simulink model "purePursuit2"  (R2022a)
settings: Solver=VariableStepAuto  StartTime=0.0  StopTime=inf  RelTol=1e-3
undefined symbols (not defined in the file or in its folder): Angular, esc, hz, L, ld, Linear, path
libraries: robotlib x3, dspstat3 x1
settings Model: Creator=kisho  LastModifiedBy=kishor
settings DebuggingCC: UnconnectedInputMsg=warning  UnconnectedOutputMsg=warning  UnconnectedLineMsg=warning
settings RTWCC: DLArmComputeVersion=19.05

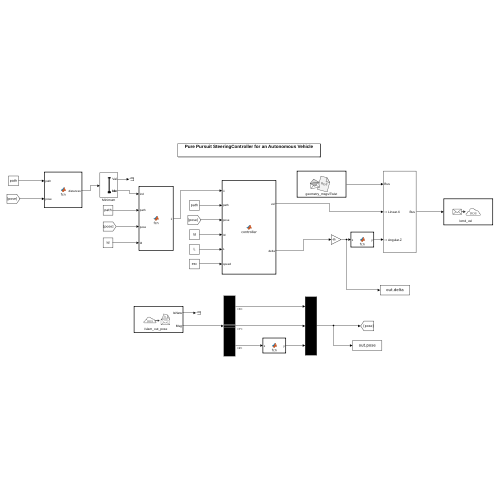
[thumbnail: Simulink's stored preview of the top-level diagram]
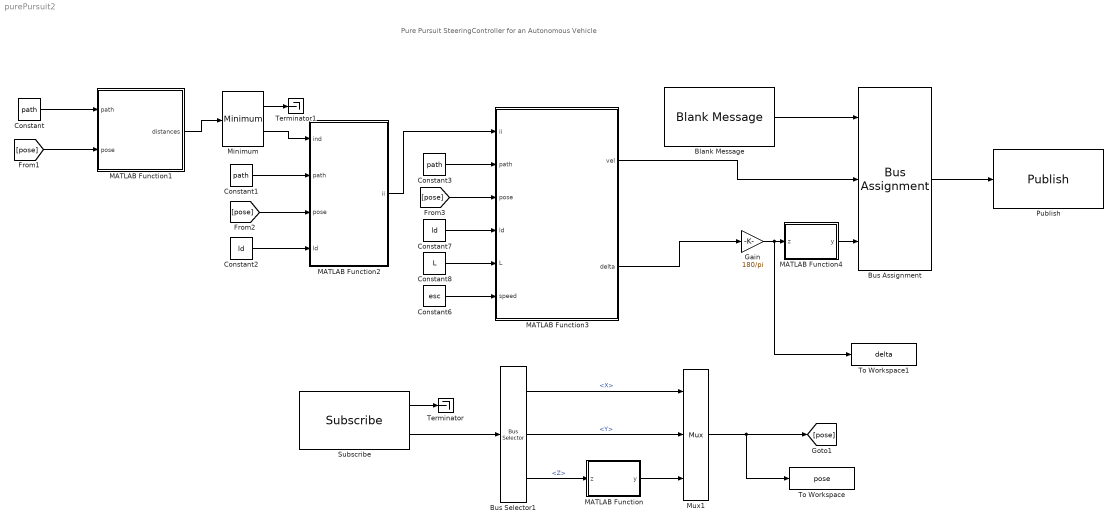
== system purePursuit2 ==
  note: Pure Pursuit SteeringController for an Autonomous Vehicle
  Blank Message : robotlib/Blank Message  messageClass=Message  entityType=geometry_msgs/Twist  messageType=geometry_msgs/Twist  SampleTime=1/hz  legacyBusStruct=off
  Bus Assignment : BusAssignment  AssignedSignals=Linear.X,Angular.Z
  Bus Selector1 : BusSelector  OutputSignals=Pose.Position.X,Pose.Position.Y,Pose.Orientation.Z
  Constant : Constant  Value=path  SampleTime=1/hz
  Constant1 : Constant  Value=path  SampleTime=1/hz
  Constant2 : Constant  Value=ld  SampleTime=1/hz
  Constant3 : Constant  Value=path  SampleTime=1/hz
  Constant6 : Constant  Value=esc  SampleTime=1/hz
  Constant7 : Constant  Value=ld  SampleTime=1/hz
  Constant8 : Constant  Value=L  SampleTime=1/hz
  Gain : Gain  Gain=180/pi
  MATLAB Function : MATLAB Function  TreatAsAtomicUnit=on
  MATLAB Function1 : MATLAB Function  TreatAsAtomicUnit=on
  MATLAB Function2 : MATLAB Function  TreatAsAtomicUnit=on
  MATLAB Function3 : MATLAB Function  TreatAsAtomicUnit=on
  MATLAB Function4 : MATLAB Function  TreatAsAtomicUnit=on
  Minimum : dspstat3/Minimum  operation=minimum  fcn=Value and Index  indexBase=One  operateOver=Each row  Dimension=1  InputProcessing=Columns as channels (frame based)  reset=None  roiEnable=off  roiType=Rectangles  roiPortion=Entire ROI  roiOutput=Individual statistics for each ROI  roiFlag=off  roundingMode=Floor  overflowMode=off
  Mux1 : Mux  Inputs=3
  Publish : robotlib/Publish  topicSource=Specify your own  topic=/cmd_vel  messageType=geometry_msgs/Twist  legacyBusStruct=off  messageQueueLength=1
  Subscribe : robotlib/Subscribe  topicSource=Specify your own  topic=/slam_out_pose  messageType=geometry_msgs/PoseStamped  SampleTime=1/hz  legacyBusStruct=off  messageQueueLength=1
  Terminator : Terminator
  Terminator1 : Terminator
  To Workspace : ToWorkspace  VariableName=pose  SaveFormat=Structure With Time  SampleTime=-1
  To Workspace1 : ToWorkspace  VariableName=delta  SaveFormat=Structure With Time  SampleTime=-1
  wires:
  MATLAB Function3/2(delta) -> Gain/1
  Blank Message/1 -> Bus Assignment/1
  Bus Assignment/1 -> Publish/1
  Subscribe/1 -> Terminator/1
  Subscribe/2 -> Bus Selector1/1
  Bus Selector1/1 -> Mux1/1  "<X>"
  Bus Selector1/2 -> Mux1/2  "<Y>"
  Bus Selector1/3 -> MATLAB Function/1(z)  "<Z>"
  Mux1/1 -> [pose], To Workspace/1
  MATLAB Function/1(y) -> Mux1/3
  Gain/1 -> To Workspace1/1, MATLAB Function4/1(z)
  MATLAB Function2/1(ii) -> MATLAB Function3/1(ii)
  Constant7/1 -> MATLAB Function3/4(ld)
  Constant1/1 -> MATLAB Function2/2(path)
  Constant3/1 -> MATLAB Function3/2(path)
  [pose] -> MATLAB Function3/3(pose)
  [pose] -> MATLAB Function2/3(pose)
  MATLAB Function1/1(distances) -> Minimum/1
  Minimum/2 -> MATLAB Function2/1(ind)
  Constant2/1 -> MATLAB Function2/4(ld)
  [pose] -> MATLAB Function1/2(pose)
  Constant/1 -> MATLAB Function1/1(path)
  Constant8/1 -> MATLAB Function3/5(L)
  Constant6/1 -> MATLAB Function3/6(speed)
  MATLAB Function3/1(vel) -> Bus Assignment/2
  MATLAB Function4/1(y) -> Bus Assignment/3
  Minimum/1 -> Terminator1/1

== matlab function purePursuit2/MATLAB Function1 ==
  data: path input; distances output; pose input
function distances  = fcn(path,pose)
 s = length(path);
 dx = zeros(1,s);
 dy = zeros(1,s);
 d  = zeros(1,s);
 for i = 1:s
     dx(i) = path(i,1) - pose(1);
     dy(i) = path(i,2) - pose(2);
 end
 distances = sqrt(dx.^2 + dy.^2);
end

== matlab function purePursuit2/MATLAB Function ==
  data: z input; y output
function y = fcn(z)
z = z*180;
if (z < 0)
    y = 180 + (180 + z);
else
    y = z;
end

end

== matlab function purePursuit2/MATLAB Function2 ==
  data: ind input; ii output; path input; pose input; ld input
function ii = fcn(ind,path,pose,ld)
ii = ind + 1;

dist = sqrt((path(ii,1)-pose(1))^2 + (path(ii,2)-pose(2))^2);

while (dist<ld)
    ii = ii + 1;
    dist = sqrt((path(ii,1)-pose(1))^2 + (path(ii,2)-pose(2))^2);
end

end

== matlab function purePursuit2/MATLAB Function3 ==
  data: vel output; ii input; delta output; path input; pose input; ld input; L input; speed input
function [vel,delta] = controller(ii,path,pose,ld,L,speed)

dx = path(ii,1)- pose(1);
dy = path(ii,2)- pose(2);
angle = atan2d(dy,dx);
if(angle < 180)
    angle = 180 + (180 +angle);
else
end

alpha = (angle - pose(3))*pi/180;

k = 2*sin(alpha)/ld;
delta = atan(k*L);

if (ii>length(path))
    vel = 0;
    delta = 0;
   
else
    vel=speed;


end

== matlab function purePursuit2/MATLAB Function4 ==
  data: z input; y output
function y = fcn(z)

if (z > 25)
    z = 25;
elseif (z < -25)
    z = -25;
else
    z =z;
end

y = z;
end
